simulink model "quadruped2"  (R2019b)
settings: Solver=FixedStepAuto  StartTime=0.0  StopTime=10.0  FixedStep=0.001  RelTol=1e-3
values from neighbouring files (symbols this model uses):
  m = sum(ml1)    [parameter_file.m]
undefined symbols (not defined in the file or in its folder): X, Y, Z
libraries: sm_lib x74, nesl_utility x18, Contact_Forces_Lib x5, sharedtransform x1
(part 3 of 3)

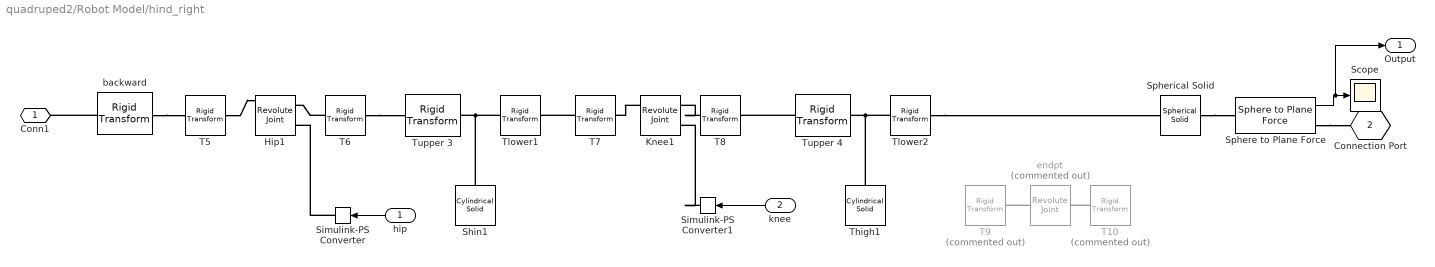
== system quadruped2/Robot Model/hind_right ==
  hip : Inport
  knee : Inport  Port=2
  Hip1 : sm_lib/Joints/Revolute Joint  JointMode=Normal  SenseConstraintForce=off  SenseConstraintForceX=off  SenseConstraintForceY=off  SenseConstraintForceZ=off  SenseConstraintTorque=off  SenseConstraintTorqueX=off  SenseConstraintTorqueY=off  SenseConstraintTorqueZ=off  SenseTotalForce=off  SenseTotalForceX=off  SenseTotalForceY=off  SenseTotalForceZ=off  SenseTotalTorque=off  SenseTotalTorqueX=off  SenseTotalTorqueY=off  SenseTotalTorqueZ=off  CompositeWrenchDir=FollowerOnBase  CompositeWrenchFrame=BaseFrame  EquilibriumPosition=0  EquilibriumPositionUnits=deg  SpringStiffness=0  SpringStiffnessUnits=N*m/deg  DampingCoefficient=0  DampingCoefficientUnits=N*m/(deg/s)  TorqueActuationMode=ComputedTorque  MotionActuationMode=InputMotion  SensePosition=on  SenseVelocity=off  SenseAcceleration=off  SenseTorqueForce=on  SenseLowerLimitTorqueForce=off  SenseUpperLimitTorqueForce=off  LowerLimitSpecify=off  LowerLimitBound=-90  LowerLimitBoundUnits=deg  LowerLimitStiffness=1e4  LowerLimitStiffnessUnits=N*m/deg  LowerLimitDamping=10  LowerLimitDampingUnits=N*m/(deg/s)  LowerLimitTransitionRegionWidth=0.1  LowerLimitTransitionRegionWidthUnits=deg  UpperLimitSpecify=off  UpperLimitBound=90  UpperLimitBoundUnits=deg  UpperLimitStiffness=1e4  UpperLimitStiffnessUnits=N*m/deg  UpperLimitDamping=10  UpperLimitDampingUnits=N*m/(deg/s)  UpperLimitTransitionRegionWidth=0.1  UpperLimitTransitionRegionWidthUnits=deg  PositionTargetSpecify=on  PositionTargetPriority=High  PositionTargetValue=30  PositionTargetValueUnits=deg  VelocityTargetSpecify=off  VelocityTargetPriority=High  VelocityTargetValue=0  VelocityTargetValueUnits=deg/s
  Knee1 : sm_lib/Joints/Revolute Joint  JointMode=Normal  SenseConstraintForce=off  SenseConstraintForceX=off  SenseConstraintForceY=off  SenseConstraintForceZ=off  SenseConstraintTorque=off  SenseConstraintTorqueX=off  SenseConstraintTorqueY=off  SenseConstraintTorqueZ=off  SenseTotalForce=off  SenseTotalForceX=off  SenseTotalForceY=off  SenseTotalForceZ=off  SenseTotalTorque=off  SenseTotalTorqueX=off  SenseTotalTorqueY=off  SenseTotalTorqueZ=off  CompositeWrenchDir=FollowerOnBase  CompositeWrenchFrame=BaseFrame  EquilibriumPosition=0  EquilibriumPositionUnits=deg  SpringStiffness=0  SpringStiffnessUnits=N*m/deg  DampingCoefficient=0  DampingCoefficientUnits=N*m/(deg/s)  TorqueActuationMode=ComputedTorque  MotionActuationMode=InputMotion  SensePosition=on  SenseVelocity=off  SenseAcceleration=off  SenseTorqueForce=off  SenseLowerLimitTorqueForce=off  SenseUpperLimitTorqueForce=off  LowerLimitSpecify=off  LowerLimitBound=-90  LowerLimitBoundUnits=deg  LowerLimitStiffness=1e4  LowerLimitStiffnessUnits=N*m/deg  LowerLimitDamping=10  LowerLimitDampingUnits=N*m/(deg/s)  LowerLimitTransitionRegionWidth=0.1  LowerLimitTransitionRegionWidthUnits=deg  UpperLimitSpecify=off  UpperLimitBound=90  UpperLimitBoundUnits=deg  UpperLimitStiffness=1e4  UpperLimitStiffnessUnits=N*m/deg  UpperLimitDamping=10  UpperLimitDampingUnits=N*m/(deg/s)  UpperLimitTransitionRegionWidth=0.1  UpperLimitTransitionRegionWidthUnits=deg  PositionTargetSpecify=on  PositionTargetPriority=High  PositionTargetValue=-60  PositionTargetValueUnits=deg  VelocityTargetSpecify=off  VelocityTargetPriority=High  VelocityTargetValue=0  VelocityTargetValueUnits=deg/s
  Scope : Scope
  Shin1 : sm_lib/Body Elements/Cylindrical Solid  GraphicAmbientColor=[0.15 0.15 0.15 1.0]  BasedOnType=Mass  CenterOfMass=[0 0 0]  CenterOfMassUnits=m  GraphicDiffuseColor=[0.5 0.5 0.5]  CylinderLength=6  CylinderLengthUnits=cm  CylinderRadius=1  CylinderRadiusUnits=cm  Density=2000  DensityUnits=kg/m^3  DoExposeReferenceFrame=on  GraphicEmissiveColor=[0.0 0.0 0.0 1.0]  ExportEntireGeometry=off  SerializedFrames=<Frames/>  MarkerShape=Sphere  MarkerSize=10  GraphicType=FromGeometry  InertiaType=CalculateFromGeometry  Mass=0.3  MassUnits=kg  MomentsOfInertia=[1 1 1]  MomentsOfInertiaUnits=kg*m^2  GraphicOpacity=1.0  ProductsOfInertia=[0 0 0]  ProductsOfInertiaUnits=kg*m^2  GraphicShininess=75  GraphicSpecularColor=[0.5 0.5 0.5 1.0]  GraphicVisPropType=SimpleVisualProperties
  Simulink-PS Converter : nesl_utility/Simulink-PS Converter  PhysicalDomain=network_engine_domain  SubClassName=ps_input  LeftPortType=input  RightPortType=output  PseudoPeriodic=off  Frequencies=[]  NoiseDistribution=none  NoiseParameters=[]  Unit=deg  AffineConversion=off  FilteringAndDerivatives=filter  SimscapeFilterOrder=2  InputFilterTimeConstant=0.001  UdotUserProvided=0
  Simulink-PS Converter1 : nesl_utility/Simulink-PS Converter  PhysicalDomain=network_engine_domain  SubClassName=ps_input  LeftPortType=input  RightPortType=output  PseudoPeriodic=off  Frequencies=[]  NoiseDistribution=none  NoiseParameters=[]  Unit=deg  AffineConversion=off  FilteringAndDerivatives=filter  SimscapeFilterOrder=2  InputFilterTimeConstant=0.001  UdotUserProvided=0
  Sphere to Plane Force : Contact_Forces_Lib/3D/Sphere to Plane Force  sphere_rad=0.0075  plane_lenx=5  plane_leny=5  plane_depth=0.5  force_law=Linear  k_contact=1e4  b_contact=1e2  pen_full_damp_F=1e-4  pen_exponent=1  custom_param_1=1  custom_param_2=1  friction_law=Stick-Slip Continuous  mu_kinetic=0.8  mu_static=0.9  v_thr=0.001  vis_on=off  vis_opc_en=0  vis_len_plaBz=0.005  vis_clr=[0.9 0.2 0.2]  vis_opc=0.7
  Spherical Solid : sm_lib/Body Elements/Spherical Solid  GraphicAmbientColor=[0.15 0.15 0.15 1.0]  BasedOnType=Density  CenterOfMass=[0 0 0]  CenterOfMassUnits=m  GraphicDiffuseColor=[0.5 0.5 0.5]  Density=1000  DensityUnits=kg/m^3  DoExposeReferenceFrame=on  GraphicEmissiveColor=[0.0 0.0 0.0 1.0]  ExportEntireGeometry=off  SerializedExposedGeometries=<ExposedGeometries/>  SerializedFrames=<Frames><Frame><Id>Frame1</Id><Value><Name>F1</Name><Origin><Source>GeometricFeature</Source><FeatureName>spherical surface</FeatureName></Origin><PrimaryAxis><DefinedDirection>+Z</DefinedDirection><Source>ReferenceFrame</Source><SourceDirection>+Z</SourceDirection><FeatureName></FeatureName></PrimaryAxis><SecondaryAxis><DefinedDirection>+X</DefinedDirection><Source>ReferenceFrame</Source><SourceDirection>+X</SourceDirection><FeatureName></FeatureName></SecondaryAxis></Value></Frame></Frames>  MarkerShape=Sphere  MarkerSize=10  GraphicType=FromGeometry  InertiaType=CalculateFromGeometry  Mass=1  MassUnits=kg  MomentsOfInertia=[1 1 1]  MomentsOfInertiaUnits=kg*m^2  GraphicOpacity=1.0  ProductsOfInertia=[0 0 0]  ProductsOfInertiaUnits=kg*m^2  GraphicShininess=75  GraphicSpecularColor=[0.5 0.5 0.5 1.0]  SphereRadius=0.75  SphereRadiusUnits=cm  GraphicVisPropType=SimpleVisualProperties
      settings: SourceProductName=Simscape Multibody
  T10 : sm_lib/Frames and Transforms/Rigid Transform  Commented=on  TranslationMethod=None  TranslationStandardOffset=90  TranslationLengthUnit=cm  TranslationStandardAxis=+X  TranslationCartesianOffset=[0 4 0]  TranslationROffset=0  TranslationROffsetUnits=m  TranslationZOffset=0  TranslationZOffsetUnits=m  TranslationThetaOffset=0  TranslationThetaOffsetUnits=deg  RotationMethod=StandardAxis  RotationAngleUnits=deg  RotationStandardAxis=+X  RotationAngle=90  RotationArbitraryAxis=[0 0 1]  FollAlignAxisA=+X  BaseAlignAxisA=+Y  FollAlignAxisB=+Y  BaseAlignAxisB=+Z  RotationSequenceAxes=FollowerAxes  RotationSequence=XYX  RotationSequenceAngles=[0 0 0]  RotationSequenceAnglesUnits=deg  RotationMatrix=[1 0 0; 0 1 0; 0 0 1]
  T5 : sm_lib/Frames and Transforms/Rigid Transform  TranslationMethod=None  TranslationStandardOffset=90  TranslationLengthUnit=cm  TranslationStandardAxis=+X  TranslationCartesianOffset=[0 4 0]  TranslationROffset=0  TranslationROffsetUnits=m  TranslationZOffset=0  TranslationZOffsetUnits=m  TranslationThetaOffset=0  TranslationThetaOffsetUnits=deg  RotationMethod=StandardAxis  RotationAngleUnits=deg  RotationStandardAxis=-X  RotationAngle=90  RotationArbitraryAxis=[0 0 1]  FollAlignAxisA=+X  BaseAlignAxisA=+Y  FollAlignAxisB=+Y  BaseAlignAxisB=+Z  RotationSequenceAxes=FollowerAxes  RotationSequence=XYX  RotationSequenceAngles=[0 0 0]  RotationSequenceAnglesUnits=deg  RotationMatrix=[1 0 0; 0 1 0; 0 0 1]
  T6 : sm_lib/Frames and Transforms/Rigid Transform  TranslationMethod=None  TranslationStandardOffset=90  TranslationLengthUnit=cm  TranslationStandardAxis=+X  TranslationCartesianOffset=[0 4 0]  TranslationROffset=0  TranslationROffsetUnits=m  TranslationZOffset=0  TranslationZOffsetUnits=m  TranslationThetaOffset=0  TranslationThetaOffsetUnits=deg  RotationMethod=StandardAxis  RotationAngleUnits=deg  RotationStandardAxis=+X  RotationAngle=90  RotationArbitraryAxis=[0 0 1]  FollAlignAxisA=+X  BaseAlignAxisA=+Y  FollAlignAxisB=+Y  BaseAlignAxisB=+Z  RotationSequenceAxes=FollowerAxes  RotationSequence=XYX  RotationSequenceAngles=[0 0 0]  RotationSequenceAnglesUnits=deg  RotationMatrix=[1 0 0; 0 1 0; 0 0 1]
  T7 : sm_lib/Frames and Transforms/Rigid Transform  TranslationMethod=None  TranslationStandardOffset=90  TranslationLengthUnit=cm  TranslationStandardAxis=+X  TranslationCartesianOffset=[0 4 0]  TranslationROffset=0  TranslationROffsetUnits=m  TranslationZOffset=0  TranslationZOffsetUnits=m  TranslationThetaOffset=0  TranslationThetaOffsetUnits=deg  RotationMethod=StandardAxis  RotationAngleUnits=deg  RotationStandardAxis=-X  RotationAngle=90  RotationArbitraryAxis=[0 0 1]  FollAlignAxisA=+X  BaseAlignAxisA=+Y  FollAlignAxisB=+Y  BaseAlignAxisB=+Z  RotationSequenceAxes=FollowerAxes  RotationSequence=XYX  RotationSequenceAngles=[0 0 0]  RotationSequenceAnglesUnits=deg  RotationMatrix=[1 0 0; 0 1 0; 0 0 1]
  T8 : sm_lib/Frames and Transforms/Rigid Transform  TranslationMethod=None  TranslationStandardOffset=90  TranslationLengthUnit=cm  TranslationStandardAxis=+X  TranslationCartesianOffset=[0 4 0]  TranslationROffset=0  TranslationROffsetUnits=m  TranslationZOffset=0  TranslationZOffsetUnits=m  TranslationThetaOffset=0  TranslationThetaOffsetUnits=deg  RotationMethod=StandardAxis  RotationAngleUnits=deg  RotationStandardAxis=+X  RotationAngle=90  RotationArbitraryAxis=[0 0 1]  FollAlignAxisA=+X  BaseAlignAxisA=+Y  FollAlignAxisB=+Y  BaseAlignAxisB=+Z  RotationSequenceAxes=FollowerAxes  RotationSequence=XYX  RotationSequenceAngles=[0 0 0]  RotationSequenceAnglesUnits=deg  RotationMatrix=[1 0 0; 0 1 0; 0 0 1]
  T9 : sm_lib/Frames and Transforms/Rigid Transform  Commented=on  TranslationMethod=None  TranslationStandardOffset=90  TranslationLengthUnit=cm  TranslationStandardAxis=+X  TranslationCartesianOffset=[0 4 0]  TranslationROffset=0  TranslationROffsetUnits=m  TranslationZOffset=0  TranslationZOffsetUnits=m  TranslationThetaOffset=0  TranslationThetaOffsetUnits=deg  RotationMethod=StandardAxis  RotationAngleUnits=deg  RotationStandardAxis=-X  RotationAngle=90  RotationArbitraryAxis=[0 0 1]  FollAlignAxisA=+X  BaseAlignAxisA=+Y  FollAlignAxisB=+Y  BaseAlignAxisB=+Z  RotationSequenceAxes=FollowerAxes  RotationSequence=XYX  RotationSequenceAngles=[0 0 0]  RotationSequenceAnglesUnits=deg  RotationMatrix=[1 0 0; 0 1 0; 0 0 1]
  Thigh1 : sm_lib/Body Elements/Cylindrical Solid  GraphicAmbientColor=[0.15 0.15 0.15 1.0]  BasedOnType=Mass  CenterOfMass=[0 0 0]  CenterOfMassUnits=m  GraphicDiffuseColor=[0.5 0.5 0.5]  CylinderLength=8  CylinderLengthUnits=cm  CylinderRadius=1  CylinderRadiusUnits=cm  Density=2000  DensityUnits=kg/m^3  DoExposeReferenceFrame=on  GraphicEmissiveColor=[0.0 0.0 0.0 1.0]  ExportEntireGeometry=off  SerializedFrames=<Frames/>  MarkerShape=Sphere  MarkerSize=10  GraphicType=FromGeometry  InertiaType=CalculateFromGeometry  Mass=0.3  MassUnits=kg  MomentsOfInertia=[1 1 1]  MomentsOfInertiaUnits=kg*m^2  GraphicOpacity=1.0  ProductsOfInertia=[0 0 0]  ProductsOfInertiaUnits=kg*m^2  GraphicShininess=75  GraphicSpecularColor=[0.5 0.5 0.5 1.0]  GraphicVisPropType=SimpleVisualProperties
  Tlower1 : sm_lib/Frames and Transforms/Rigid Transform  TranslationMethod=StandardAxis  TranslationStandardOffset=3  TranslationLengthUnit=cm  TranslationStandardAxis=+Z  TranslationCartesianOffset=[0 0 0]  TranslationROffset=0  TranslationROffsetUnits=m  TranslationZOffset=0  TranslationZOffsetUnits=m  TranslationThetaOffset=0  TranslationThetaOffsetUnits=deg  RotationMethod=None  RotationAngleUnits=deg  RotationStandardAxis=+X  RotationAngle=90  RotationArbitraryAxis=[0 0 1]  FollAlignAxisA=+X  BaseAlignAxisA=+Y  FollAlignAxisB=+Y  BaseAlignAxisB=+Z  RotationSequenceAxes=FollowerAxes  RotationSequence=XYX  RotationSequenceAngles=[0 0 0]  RotationSequenceAnglesUnits=deg  RotationMatrix=[1 0 0; 0 1 0; 0 0 1]
  Tlower2 : sm_lib/Frames and Transforms/Rigid Transform  TranslationMethod=StandardAxis  TranslationStandardOffset=4  TranslationLengthUnit=cm  TranslationStandardAxis=+Z  TranslationCartesianOffset=[0 0 0]  TranslationROffset=0  TranslationROffsetUnits=m  TranslationZOffset=0  TranslationZOffsetUnits=m  TranslationThetaOffset=0  TranslationThetaOffsetUnits=deg  RotationMethod=None  RotationAngleUnits=deg  RotationStandardAxis=+X  RotationAngle=90  RotationArbitraryAxis=[0 0 1]  FollAlignAxisA=+X  BaseAlignAxisA=+Y  FollAlignAxisB=+Y  BaseAlignAxisB=+Z  RotationSequenceAxes=FollowerAxes  RotationSequence=XYX  RotationSequenceAngles=[0 0 0]  RotationSequenceAnglesUnits=deg  RotationMatrix=[1 0 0; 0 1 0; 0 0 1]
  Tupper 3 : sm_lib/Frames and Transforms/Rigid Transform  TranslationMethod=StandardAxis  TranslationStandardOffset=3  TranslationLengthUnit=cm  TranslationStandardAxis=+Z  TranslationCartesianOffset="[18  10 4]"  TranslationROffset=0  TranslationROffsetUnits=m  TranslationZOffset=0  TranslationZOffsetUnits=m  TranslationThetaOffset=0  TranslationThetaOffsetUnits=deg  RotationMethod=None  RotationAngleUnits=deg  RotationStandardAxis=+X  RotationAngle=90  RotationArbitraryAxis=[0 0 1]  FollAlignAxisA=+X  BaseAlignAxisA=+Y  FollAlignAxisB=+Y  BaseAlignAxisB=+Z  RotationSequenceAxes=FollowerAxes  RotationSequence=XYX  RotationSequenceAngles=[0 0 0]  RotationSequenceAnglesUnits=deg  RotationMatrix=[1 0 0; 0 1 0; 0 0 1]
  Tupper 4 : sm_lib/Frames and Transforms/Rigid Transform  TranslationMethod=StandardAxis  TranslationStandardOffset=4  TranslationLengthUnit=cm  TranslationStandardAxis=+Z  TranslationCartesianOffset="[18  10 4]"  TranslationROffset=0  TranslationROffsetUnits=m  TranslationZOffset=0  TranslationZOffsetUnits=m  TranslationThetaOffset=0  TranslationThetaOffsetUnits=deg  RotationMethod=None  RotationAngleUnits=deg  RotationStandardAxis=+X  RotationAngle=90  RotationArbitraryAxis=[0 0 1]  FollAlignAxisA=+X  BaseAlignAxisA=+Y  FollAlignAxisB=+Y  BaseAlignAxisB=+Z  RotationSequenceAxes=FollowerAxes  RotationSequence=XYX  RotationSequenceAngles=[0 0 0]  RotationSequenceAnglesUnits=deg  RotationMatrix=[1 0 0; 0 1 0; 0 0 1]
  backward : sm_lib/Frames and Transforms/Rigid Transform  TranslationMethod=Cartesian  TranslationStandardOffset=4  TranslationLengthUnit=cm  TranslationStandardAxis=+Z  TranslationCartesianOffset=[17 10 0]  TranslationROffset=0  TranslationROffsetUnits=m  TranslationZOffset=0  TranslationZOffsetUnits=m  TranslationThetaOffset=0  TranslationThetaOffsetUnits=deg  RotationMethod=None  RotationAngleUnits=deg  RotationStandardAxis=+X  RotationAngle=90  RotationArbitraryAxis=[0 0 1]  FollAlignAxisA=+X  BaseAlignAxisA=+Y  FollAlignAxisB=+Y  BaseAlignAxisB=+Z  RotationSequenceAxes=FollowerAxes  RotationSequence=XYX  RotationSequenceAngles=[0 0 0]  RotationSequenceAnglesUnits=deg  RotationMatrix=[1 0 0; 0 1 0; 0 0 1]
  endpt : sm_lib/Joints/Revolute Joint  Commented=on  JointMode=Normal  SenseConstraintForce=off  SenseConstraintForceX=off  SenseConstraintForceY=off  SenseConstraintForceZ=off  SenseConstraintTorque=off  SenseConstraintTorqueX=off  SenseConstraintTorqueY=off  SenseConstraintTorqueZ=off  SenseTotalForce=off  SenseTotalForceX=off  SenseTotalForceY=off  SenseTotalForceZ=off  SenseTotalTorque=off  SenseTotalTorqueX=off  SenseTotalTorqueY=off  SenseTotalTorqueZ=off  CompositeWrenchDir=FollowerOnBase  CompositeWrenchFrame=BaseFrame  EquilibriumPosition=0  EquilibriumPositionUnits=deg  SpringStiffness=0  SpringStiffnessUnits=N*m/deg  DampingCoefficient=0  DampingCoefficientUnits=N*m/(deg/s)  TorqueActuationMode=NoTorque  MotionActuationMode=ComputedMotion  SensePosition=off  SenseVelocity=off  SenseAcceleration=off  SenseTorqueForce=off  SenseLowerLimitTorqueForce=off  SenseUpperLimitTorqueForce=off  LowerLimitSpecify=off  LowerLimitBound=-90  LowerLimitBoundUnits=deg  LowerLimitStiffness=1e4  LowerLimitStiffnessUnits=N*m/deg  LowerLimitDamping=10  LowerLimitDampingUnits=N*m/(deg/s)  LowerLimitTransitionRegionWidth=0.1  LowerLimitTransitionRegionWidthUnits=deg  UpperLimitSpecify=off  UpperLimitBound=90  UpperLimitBoundUnits=deg  UpperLimitStiffness=1e4  UpperLimitStiffnessUnits=N*m/deg  UpperLimitDamping=10  UpperLimitDampingUnits=N*m/(deg/s)  UpperLimitTransitionRegionWidth=0.1  UpperLimitTransitionRegionWidthUnits=deg  PositionTargetSpecify=off  PositionTargetPriority=High  PositionTargetValue=0  PositionTargetValueUnits=deg  VelocityTargetSpecify=off  VelocityTargetPriority=High  VelocityTargetValue=0  VelocityTargetValueUnits=deg/s
  Conn1 : PMIOPort  Side=Left
  Connection Port : PMIOPort  Tag=PMCPort  Port=2  Side=Left
  Output : Outport
  wires:
  Sphere to Plane Force/1 -> Output/1, Scope/1
  hip/1 -> Simulink-PS Converter/1
  knee/1 -> Simulink-PS Converter1/1
  connections:
  Spherical Solid/LConn1 -- Sphere to Plane Force/LConn1
  Sphere to Plane Force/RConn1 -- Connection Port/RConn1
  endpt/RConn1 -- T9/LConn1
  T10/RConn1 -- endpt/LConn1
  T6/RConn1 -- Hip1/LConn1
  T8/RConn1 -- Knee1/LConn1
  backward/RConn1 -- Conn1/RConn1
  T6/LConn1 -- Tupper 3/RConn1
  Tupper 4/LConn1 -- Tlower2/RConn1 -- Thigh1/RConn1
  Tupper 4/RConn1 -- T8/LConn1
  T7/RConn1 -- Tlower1/LConn1
  Tupper 3/LConn1 -- Tlower1/RConn1 -- Shin1/RConn1
  Knee1/RConn1 -- T7/LConn1
  T5/LConn1 -- Hip1/RConn1
  backward/LConn1 -- T5/RConn1
  Simulink-PS Converter/RConn1 -- Hip1/LConn2
  Simulink-PS Converter1/RConn1 -- Knee1/LConn2
  Tlower2/LConn1 -- Spherical Solid/RConn1

== matlab function quadruped2/Reference Trajectory Generation ==
  data: Xref2 output; X input; Xref output
function [Xref2,Xref] = Ref_Trajectory(X)
    
    Tm = 0.4;   % Swing Phase Period
    Ts = 0.4;   % Stance Phase Period
    S = 2.0; %cm  Stride length
    H = 1.0; %cm   Stride Height
    T = 0.8;
    dt = 0.001;

    k=0.1; % Scaling Factor

   
    oy=-11; %cm
    ox = -S/2;

    alpha = 50;
    b = 50;
    gamma = 50;
    beta = 0.5; % for trot; for walk beta = 0.75
    delta = 0.3; %for trot; for walk delta = 1
    meu1 = 1;
    meu2 = 1;

     R = [1 0 -1 0 1 0 -1 0
         0 1 0 -1 0 1 0 -1
         -1 0 1 0 -1 0 1 0
         0 -1 0 1 0 -1 0 1
         1 0 -1 0 1 0 -1 0
         0 1 0 -1 0 1 0 -1
         -1 0 1 0 -1 0 1 0
         0 -1 0 1 0 -1 0 1];
     
     x2 = X;

     C = eye(8);

    %          R = [1 0 -1 0 0 1 0 -1
    %               0 1 0 -1 -1 0 1 0
    %               -1 0 1 0 0 -1 0 1
    %               0 -1 0 1 1 0 -1 0
    %               0 -1 0 1 1 0 -1 0
    %               1 0 -1 0 0 1 0 -1 
    %               0 1 0 -1 -1 0 1 0 
    %               -1 0 1 0 0 -1 0 1];
    %          delta = 1; beta=0.75;
    
    %          R = [1 0 -1 0 1 0 -1 0
    %              0 1 0 -1 0 1 0 -1
    %              -1 0 1 0 -1 0 1 0
    %              0 -1 0 1 0 -1 0 1
    %              1 0 -1 0 1 0 -1 0
    %              0 1 0 -1 0 1 0 -1
    %              -1 0 1 0 -1 0 1 0
    %              0 -1 0 1 0 -1 0 1];
    %          delta = 0.3;beta = 0.5;
    
    r1 = sqrt(x2(1)^2 + x2(2)^2);
    r2 = sqrt(x2(3)^2 + x2(4)^2);
    r3 = sqrt(x2(5)^2 + x2(6)^2);
    r4 = sqrt(x2(7)^2 + x2(8)^2);
    w1 = pi/(beta*T*(exp(-b*x2(2))+1)) + pi/((1-beta)*T*(exp(b*x2(2))+1));
    w2 = pi/(beta*T*(exp(-b*x2(4))+1)) + pi/((1-beta)*T*(exp(b*x2(4))+1));
    w3 = pi/(beta*T*(exp(-b*x2(6))+1)) + pi/((1-beta)*T*(exp(b*x2(6))+1));
    w4 = pi/(beta*T*(exp(-b*x2(8))+1)) + pi/((1-beta)*T*(exp(b*x2(8))+1));
    A = [alpha*(meu1-r1^2) -w1 0 0 0 0 0 0
          w1 gamma*(meu1-r1^2) 0 0 0 0 0 0
          0 0 alpha*(meu2-r2^2) -w2 0 0 0 0
          0 0 w2 gamma*(meu2-r2^2) 0 0 0 0
          0 0 0 0 alpha*(meu1-r3^2) -w3 0 0 
          0 0 0 0 w3 gamma*(meu1-r3^2) 0 0
          0 0 0 0 0 0 alpha*(meu2-r4^2) -w4
          0 0 0 0 0 0 w4 gamma*(meu2-r4^2)];
    B = delta*R;
    v = A*x2 + B*x2;
    Xref2 = x2 + dt*v;

    Xref = Xref2;
    
    Xref(2) = H*Xref(2).*(Xref(2)>=0) + oy;
    Xref(4) = H*Xref(4).*(Xref(4)>=0) + oy;
    Xref(6) = H*Xref(6).*(Xref(6)>=0) + oy;
    Xref(8) = H*Xref(8).*(Xref(8)>=0) + oy;

    Xref(1) = S*Xref(1);
    Xref(3) = S*Xref(3);
    Xref(5) = S*Xref(5);
    Xref(7) = S*Xref(7);

end

== matlab function quadruped2/MATLAB Function ==
  data: f1 input; f2 input; f3 input; f4 input; ang input; omega input; px input; py input; pz input; vx input; vy input; vz input; Xref input
function convec_MPC(f1,f2,f3,f4,ang,omega,px,py,pz,vx,vy,vz,Xref)

    yaw = 0;
    m = 7.8;
    g = 9.81;
    cl = 0.1;
    cu = 3.5;
    Ib = diag([0.018405, 0.058725, 0.07632]);
    
    f1 = [f1(2) f1(1) f1(3)]';
    f2 = [f2(2) f2(1) f2(3)]';
    f3 = [f3(2) f3(1) f3(3)]';
    f4 = [f4(2) f4(1) f4(3)]';
    
    ang = (180/pi).*ang;
    
    Rz = [cosd(yaw) sind(yaw) 0
         -sind(yaw) cosd(yaw) 0 
              0         0     1];
    r1 = [17+Xref(1),10,Xref(2)];
    r2 = [17+Xref(3),-10,Xref(4)];
    r3 = [-17+Xref(5),-10,Xref(6)];
    r4 = [-17+Xref(7),10,Xref(8)];
    
    zm = zeros(3,3);
    onem = ones(3,3);
    onem2 = [0;0;1];
    zm2 = zeros(1,3);
    zm3 = zeros(3,1);
    Iw = inv(Rz*Ib*(Rz'));
    
    
    A = [zm zm Rz zm zm3
         zm zm zm onem zm3
         zm zm zm zm zm3
         zm zm zm zm onem2
         zm2 zm2 zm2 zm2 0];
     
     r11 = [0    -r1(3) r1(2)
            r1(3)   0  -r1(1)
           -r1(2) r1(1)  0];
        
     r22 = [0    -r2(3) r2(2)
            r2(3)    0  -r2(1)
           -r2(2) r2(1)  0];
        
     r33 = [0    -r3(3)  r3(2)
            r3(3)    0   -r3(1)
           -r3(2) r3(1)  0];
        
     r44 = [0    -r4(3) r4(2)
            r4(3)  0   -r4(1)
           -r4(2) r4(1)  0];   
     
     
     B = [zm zm zm zm zm3
          zm zm zm zm zm3
          Iw*r11 Iw*r22 Iw*r33 Iw*r44 zm3
          onem./m onem./m onem./m onem./m zm3
          zm2 zm2 zm2 zm2 0];
      
     C = eye(13);
     D = zeros(13,1);

     X = [ang',px,py,pz,omega',vx,vy,vz,0]';
     Xd = [0 0 0 0 0 0 0 0 0 0 0 0 0]';
     
     U = [f1(2) f1(3) f1(1) f2(2) f2(3) f2(1) f3(2) f3(3) f3(1) f4(2) f4(3) f4(1) 0]';   % ri and fi has to a column matrix

     L = diag([1 1 1 0 0 1 0 0 1 1 1 1 0]);
     K = diag([1e-16 1e-16 1e-16 1e-16 1e-16 1e-16 1e-16 1e-16 1e-16 1e-16 1e-16 1e-16 0]);
     
     H = 2*(B'*L*B + K)
     g2 = 2*B'*L*(A*X - Xd)
     
     
     
    
end

== matlab function quadruped2/Inverse Kinematics  ==
  data: theta output; X input; t11 output; t12 output; t21 output; t22 output; t31 output; t32 output; t41 output; t42 output
function [theta,t11,t12,t21,t22,t31,t32,t41,t42] = fcn(X)
    theta = zeros(8,1);
    l1=8;l2=6;
    for i=1:4
        l4 = sqrt(X(2*i-1)^2 + X(2*i)^2);
        if(X(2*i-1)>0)
            theta(2*i-1) = acosd((l4^2 + l1^2 - l1^2)/(2*l4*l1)) + abs(atand(X(2*i)/X(2*i-1))) - 90;
        else
            theta(2*i-1) = acosd((l4^2 + l1^2 - l1^2)/(2*l4*l1)) - abs(atand(X(2*i)/X(2*i-1))) + 90;
        end
        theta(2*i) = acosd((l1^2 + l2^2 - l4^2)/(2*l1*l2)) - 180;
    end
    t11 = theta(1,1);
    t12 = theta(2,1);
    
    t21 = theta(3,1);
    t22 = theta(4,1);
    
    t31 = theta(5,1);
    t32 = theta(6,1);
    
    t41 = theta(7,1);
    t42 = theta(8,1);
end
